simulink model "righthalf"  (R2018a)
settings: Solver=VariableStepAuto  StartTime=0.0  StopTime=10.0  RelTol=1e-3
undefined symbols (not defined in the file): duty
libraries: powerlib x8, powerlib_meascontrol x2, pePowerMeasurement x1, simulink x1
settings Model: Creator=DELL  LastModifiedBy=DELL

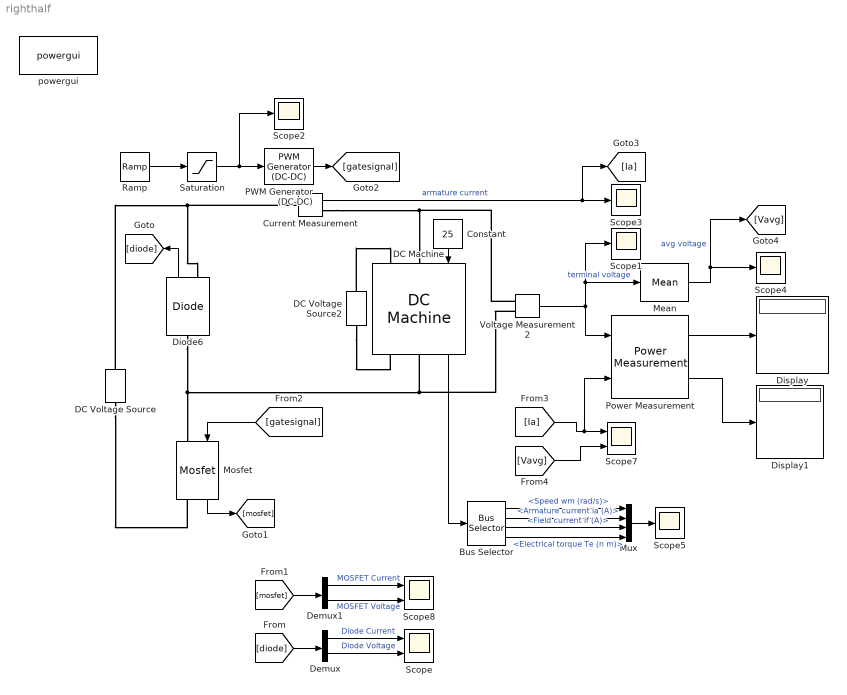
== system righthalf ==
  Bus Selector : BusSelector  OutputSignals=Speed wm (rad/s),Armature current ia (A),Field current if (A),Electrical torque Te (n m)
  Constant : Constant  Value=25
  Current Measurement : powerlib/Measurements/Current Measurement  PhasorSimulation=off  OutputType=Complex  PSBequivalent=0
  DC Machine : powerlib/Machines/DC Machine  PresetModel=No  MechanicalLoad=Torque TL  FieldType=Wound  ShowDetailedParameters=on  MeasurementBus=off  RLa="[ 1.07  0.0245]"  RLf="[ 210  23]"  Laf=1.8  MachineConstant=Torque constant (N.m/A)  Ke=1.8  Kt=1.8  J=1  Bm=0  Tf=0  w0=1  Ifinit=1  TsPowergui=0  TsBlock=-1
  DC Voltage Source : powerlib/Electrical Sources/DC Voltage Source  Amplitude=160  Measurements=None
  DC Voltage Source2 : powerlib/Electrical Sources/DC Voltage Source  Amplitude=220  Measurements=None
  Demux : Demux  Outputs=2
  Demux1 : Demux  Outputs=2
  Diode6 : powerlib/Power Electronics/Diode  Ron=0.001  Lon=0  Vf=1.5  IC=0  UseSnubber=off  Rs=inf  Cs=0  Measurements=on
  Display : Display
  Display1 : Display
  Mean : powerlib_meascontrol/Measurements/Mean  Freq=60  Vinit=0  Ts=0
  Mosfet : powerlib/Power Electronics/Mosfet  Ron=0.085  Lon=0  Rd=0.01  Vfd=0  IC=0  Rs=1e5  Cs=inf  Measurements=on
  Mux : Mux
  PWM Generator (DC-DC) : powerlib_meascontrol/Pulse & Signal Generators/PWM Generator (DC-DC)  Fsw=20000  Ts=0
  Power Measurement : pePowerMeasurement/Power Measurement  OverrideUsingVariant=Continuous  F=60  K=[0 1 2 3]  Ts=0
  Ramp : simulink/Sources/Ramp  slope=duty/10  start=0  InitialOutput=0.9
  Saturation : Saturate  UpperLimit=0.9  LowerLimit=0  ZeroCross=off
  Scope : Scope  NumInputPorts=2
  Scope{1..5} (5 alike) : Scope
  Scope7 : Scope  NumInputPorts=2
  Scope8 : Scope  NumInputPorts=2
  Voltage Measurement2 : powerlib/Measurements/Voltage Measurement  PhasorSimulation=off  OutputType=Complex  PSBequivalent=0
  powergui : powerlib/powergui  Priority=1  SimulationMode=Continuous  SampleTime=50e-6  frequency=60  Iterations=50  frequencyindice=0  Pbase=100e6  ErrMax=1e-4  UnitsV=kV  UnitsW=MW  buscounter=0  FunctionMessages=off  echomessages=off  EnableUseOfTLC=off  CurrentSourceSwitches=off  DisableSnubberDevices=off  DisableRonSwitches=off  DisableVfSwitches=off  DisplayEquations=off  SolverType=Tustin/Backward Euler (TBE)  Interpol=off  ExternalGateDelay=off  methode=off  Ts=100  x0status=blocks  SPID=on  SwTol=0  HookPort=off  RestoreLinks=warning  ResistiveCurrentMeasurement=off  Frange=[0:2:500]  Ylog=off  Xlog=on  ShowGrid=off  save=off  variable=ZData  structure=0  ZoomFFT=off  StartTime=0.0  cycles=1  DisplayStyle=1  fundamental=60  FreqAxis=off  MaxFrequency=1000  frequencyindicesteady=1  RmsSteady=1  display=off
  wires:
  Mean/1 -> [Vavg], Scope4/1  "avg voltage"
  Constant/1 -> DC Machine/1
  Voltage Measurement2/1 -> Power Measurement/1, Scope1/1, Mean/1  "terminal voltage"
  Ramp/1 -> Saturation/1
  Saturation/1 -> Scope2/1, PWM Generator (DC-DC)/1
  Power Measurement/2 -> Display1/1
  Power Measurement/1 -> Display/1
  Bus Selector/3 -> Mux/3  "<Field current if (A)>"
  Bus Selector/2 -> Mux/2  "<Armature current ia (A)>"
  Mux/1 -> Scope5/1
  Bus Selector/1 -> Mux/1  "<Speed wm (rad/s)>"
  DC Machine/1 -> Bus Selector/1
  Bus Selector/4 -> Mux/4  "<Electrical torque Te (n m)>"
  Current Measurement/1 -> Scope3/1, [Ia]  "armature current"
  Diode6/1 -> [diode]
  Mosfet/1 -> [mosfet]
  PWM Generator (DC-DC)/1 -> [gatesignal]
  [gatesignal] -> Mosfet/1
  [Ia] -> Scope7/1, Power Measurement/2
  [Vavg] -> Scope7/2
  [diode] -> Demux/1
  Demux/1 -> Scope/1  "Diode Current"
  Demux/2 -> Scope/2  "Diode Voltage"
  Demux1/2 -> Scope8/2  "MOSFET Voltage"
  Demux1/1 -> Scope8/1  "MOSFET Current"
  [mosfet] -> Demux1/1
  connections:
  Diode6/LConn1 -- Mosfet/LConn1 -- Voltage Measurement2/LConn2 -- DC Machine/RConn1
  Current Measurement/RConn1 -- Voltage Measurement2/LConn1 -- DC Machine/LConn1
  DC Voltage Source2/LConn1 -- DC Machine/RConn2
  DC Voltage Source2/RConn1 -- DC Machine/LConn2
  DC Voltage Source/RConn1 -- Current Measurement/LConn1 -- Diode6/RConn1
  DC Voltage Source/LConn1 -- Mosfet/RConn1
